simulink model "SimSimulink"  (R2024a)
settings: Solver=ode4  StartTime=0.0  StopTime=Tstop  FixedStep=Ts  RelTol=1e-3
values from neighbouring files (symbols this model uses):
  Ts = 210    [SimMATLAB.m]
libraries: spsThreePhaseVIMeasurementLib x1, spsThreePhaseProgrammableVoltageSourceLib x1, spsGroundLib x1, spsAsynchronousMachinepuUnitsLib x1, sps_lib x1
settings Model: Creator=caugu  LastModifiedBy=caugu

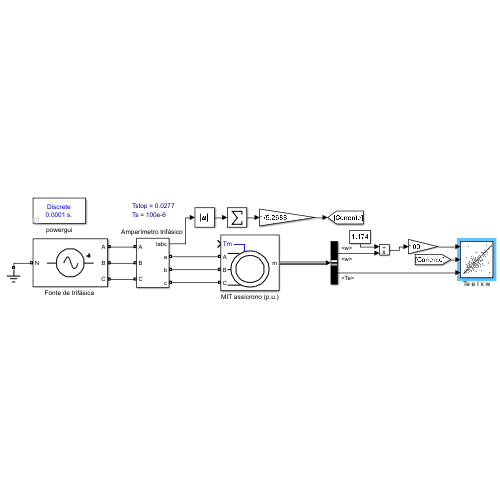
[thumbnail: Simulink's stored preview of the top-level diagram]
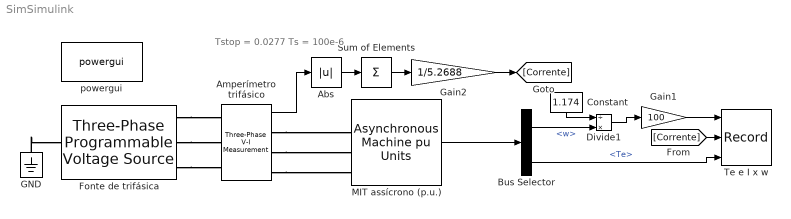
== system SimSimulink ==
  note: Tstop = 0.0277
      | Ts = 100e-6
  Abs : Abs  SaturateOnIntegerOverflow=off
  "Amperímetro trifásico " : spsThreePhaseVIMeasurementLib/Three-Phase V-I Measurement  VoltageMeasurement=no  SetLabelV=off  LabelV=Vabc  Vpu=off  VpuLL=off  CurrentMeasurement=yes  SetLabelI=off  LabelI=Iabc  Ipu=on  Pbase=746*10  Vbase=400  OutputType=Complex  PhasorSimulation=off  PSBequivalent=0
  Bus Selector : BusSelector  OutputSignals=w,Te
  Constant : Constant  Value=1.174
  Divide1 : Product  Inputs=/*
  "Fonte de trifásica " : spsThreePhaseProgrammableVoltageSourceLib/Three-Phase Programmable Voltage Source  PositiveSequence="[400  0 60]"  VariationEntity=None  VariationType=Table of time-amplitude pairs  VariationTypeAlt=Step  VariationStep=0.5  VariationRate=10  VariationMagnitude=0.3  VariationFrequency=2  VariationTiming=[1 2]  VariationPhaseA=off  Amplitudes=[1 0.8 1.2 1.0]  TimeValues=[0 0.1 0.15 0.2]  HarmonicGeneration=off  HarmonicA=[3 0.2 -25 0]  HarmonicB=[2 0.15 35 2]  Timing="[0.05  3]"  BusType=swing  Pref=0  Qref=0  Qmin=-inf  Qmax=inf
  GND : spsGroundLib/Ground  LConnTagsString=a
  Gain1 : Gain  Gain=100
  Gain2 : Gain  Gain=1/5.2688
  MIT assícrono (p.u.) : spsAsynchronousMachinepuUnitsLib/Asynchronous Machine pu Units  RotorType=Squirrel-cage  PresetModel=No  MechanicalLoad=Torque Tm  ShowDetailedParameters=on  ReferenceFrame=Rotor  Units=pu  MeasurementBus=on  NominalParameters=[746*10 400 60]  VoltageRatio=1  Stator=[0.028974 0.023606]  Rotor=[0.0192727 0.0353927]  Cage1=[0.01909 0.0397]  Cage2=[0.01909 0.0397]  Lm=1.883241938  Mechanical=[0.0455 0 3]  PolePairs=3  InitialConditions="[ 1,0,   0,0,0,  0,0,0 ]"  SimulateSaturation=off  Saturation="[0.212,0.4201,0.8125,1.0979,1.4799,2.2457,3.2586,4.5763,6.4763 ;   0.5,0.7,0.9,1,1.1,1.2 ,1.3,1.4,1.5]"  LoadFlowParameters=0  TsPowergui=0  TsBlock=-1  IterativeModel=Trapezoidal non iterative  IterativeDiscreteModel=Trapezoidal iterative (alg. loop)  Pmec=0
      settings: LibrarySourceBlock=|
      | sps_lib/Electrical Machines/Asynchronous Machine
      | pu Units
  Sum of Elements : Sum  Inputs=+
  Te e I x w : Record  FileSettingsInternal="{\"entries\":[{\"content\":{\"excelSettings\":{\"content\":{},\"type\":\"Streamout.ExcelSettings\"}},\"type\":\"Streamout.FileSettingStorage\",\"uuid\":\"\"}],\"packageUris\":[\"http:\\/\\/schema.mathworks.com\\/mf0\\/streamout_blocks\\/R2020a\"],\"version\":\"1.0\"}"  Layout=[1 1]  SignalsInternal="{\"entries\":[{\"content\":{\"signals\":[{\"content\":{\"blockPath\":[],\"dimensions\":[1],\"domain\":\"\",\"lineColor\":\"#a2142f\",\"lineWidth\":2,\"plots\":[ 1 ],\"port\":1,\"sid\":[\"\"],\"signalID\":1,\"signalName\":\"Gain1\"},\"type\":\"RecordBlkView.Signal\",\"uuid\":\"\"},{\"content\":{\"blockPath\":[],\"dimensions\":[1],\"domain\":\"\",\"lineColor\":\"#d95319\",\"lineWidth\":2,\"plots\":[ 1 ],\"port\":2,\"sid\":[\"\"],\"signalID\":2,\"signalName\":\"From\"},\"type\":\"RecordBlkView.Signal\",\"uuid\":\"\"},{\"content\":{\"blockPath\":[],\"dimensions\":[1],\"domain\":\"\",\"lineColor\":\"#b746ff\",\"lineWidth\":2,\"plots\":[ 1 ],\"port\":3,\"sid\":[\"\"],\"signalID\":3,\"signalName\":\"<Te>\"},\"type\":\"RecordBlkView.Signal\",\"uuid\":\"\"}]},\"type\":\"RecordBlkView.InputSignals\",\"uuid\":\"\"}],\"packageUris\":[\"http:\\/\\/schema.mathworks.com\\/mf0\\/streamout_blocks\\/R2020a\"],\"version\":\"1.0\"}"  VisualizationBindings="{\"xyplotplugin\":{\"info\":[{\"series\":[{\"bindingParametersList\":[{\"parameter\":\"X-Axis\",\"signalID\":1,\"signalName\":\"Gain1\"},{\"parameter\":\"Y-Axis\",\"signalID\":2,\"signalName\":\"From\"}],\"seriesID\":0},{\"bindingParametersList\":[{\"parameter\":\"X-Axis\",\"signalID\":1,\"signalName\":\"Gain1\"}],\"seriesID\":1},{\"bindingParametersList\":[{\"parameter\":\"X-Axis\",\"signalID\":1,\"signalName\":\"Gain1\"}],\"seriesID\":2},{\"bindingParametersList\":[{\"parameter\":\"X-Axis\",\"signalID\":1,\"signalName\":\"Gain1\"},{\"parameter\":\"Y-Axis\",\"signalID\":3,\"signalName\":\"<Te>\"}],\"seriesID\":3}],\"subplotID\":1}]}}"  CompatibilityTag=XY
  powergui : sps_lib/powergui  Priority=1  SimulationMode=Discrete  SampleTime=Ts  frequency=60  Iterations=50  frequencyindice=60  Pbase=100e6  ErrMax=1e-4  UnitsV=kV  UnitsW=MW  buscounter=0  FunctionMessages=off  echomessages=off  EnableUseOfTLC=off  CurrentSourceSwitches=off  DisableSnubberDevices=off  DisableRonSwitches=off  DisableVfSwitches=off  DisplayEquations=off  AutomaticDiscreteSolvers=off  SolverType=Tustin/Backward Euler (TBE)  Interpol=off  ExternalGateDelay=off  methode=off  Ts=100  x0status=blocks  SPID=on  SwTol=0  HookPort=off  NonlinearTolerance=1e-4  nMaxIteration=100  ContinueOnMaxIteration=off  RestoreLinks=warning  ResistiveCurrentMeasurement=off  Frange=[0:2:500]  Ylog=off  Xlog=on  ShowGrid=off  save=off  variable=ZData  structure=0  ZoomFFT=off  StartTime=0.0  cycles=1  DisplayStyle=1  fundamental=60  FreqAxis=off  MaxFrequency=1000  frequencyindicesteady=1  RmsSteady=1  display=off
  wires:
  Gain1/1 -> Te e I x w/1
  Sum of Elements/1 -> Gain2/1
  MIT assícrono (p.u.)/1 -> Bus Selector/1
  Divide1/1 -> Gain1/1
  Abs/1 -> Sum of Elements/1
  Bus Selector/1 -> Divide1/2  "<w>"
  "Amperímetro trifásico "/1 -> Abs/1
  Bus Selector/2 -> Te e I x w/3  "<Te>"
  Constant/1 -> Divide1/1
  Gain2/1 -> [Corrente]
  [Corrente] -> Te e I x w/2
  connections:
  "Fonte de trifásica "/RConn1 -- "Amperímetro trifásico "/LConn1
  "Amperímetro trifásico "/RConn2 -- MIT assícrono (p.u.)/LConn2
  "Fonte de trifásica "/RConn3 -- "Amperímetro trifásico "/LConn3
  GND/LConn1 -- "Fonte de trifásica "/LConn1
  "Amperímetro trifásico "/RConn3 -- MIT assícrono (p.u.)/LConn3
  "Amperímetro trifásico "/RConn1 -- MIT assícrono (p.u.)/LConn1
  "Fonte de trifásica "/RConn2 -- "Amperímetro trifásico "/LConn2
